simulink model "Robot_Eye_Control"  (R2016b)
settings: Solver=ode1  StartTime=0.0  StopTime=Inf  FixedStep=0.001  RelTol=1e-3
PostLoadFcn:
  | , if any(exist('dsrtsu_mdlpostloadfcn', 'file') == [2, 3, 6]), try dsrtsu_mdlpostloadfcn('Execute', bdroot); catch fprintf('Error in PostLoadFcn (dsrtsu_mdlpostloadfcn) for model "%s":\n %s\n', bdroot, lasterr); end, end,
libraries: simulink x4, rtiethernetlib x4, dspstat3 x3, rti1202serlib x2
settings Model: DSRTSU_INTERNAL_RTI_VER=490  DSRTSU_INTERNAL_RTI_TYPE=rti1202  DSRTSU_INTERNAL_RTIFPGA=80  Creator=labuser  LastModifiedBy=labuser
settings OptimizationCC: BlockReduction=off  ConditionallyExecuteInputs=off  OptimizeBlockIOStorage=off  BufferReuse=off  GlobalBufferReuse=off  ExpressionFolding=off  LocalBlockOutputs=off
settings HardwareCC: ProdBitPerPointer=32  ProdBitPerSizeT=32  ProdBitPerPtrDiffT=32  ProdLargestAtomicInteger=Integer  ProdEndianess=BigEndian  ProdWordSize=32  ProdHWDeviceType=Custom Processor->Custom  TargetIntDivRoundTo=Zero  TargetEndianess=BigEndian  TargetHWDeviceType=Custom Processor->Custom
settings RTWCC: SystemTargetFile=rti1202.tlc  MakeCommand=make_rti  TemplateMakefile=rti1202.tmf  Description=dSPACE DS1202 Hardware Platform
settings STFCustomTargetCC: ParMdlRefBuildCompliant=on  GRTInterface=off  SystemTargetFile=rti1202.tlc
settings GRTTargetCC: TargetLangStandard=C89/C90 (ANSI)  CompOptLevelCompliant=off  ConcurrentExecutionCompliant=off  CombineOutputUpdateFcns=off  MatFileLogging=off  CPPClassGenCompliant=off  UseToolchainInfoCompliant=off
settings ConfigComp: CovMetricSettings=dswe

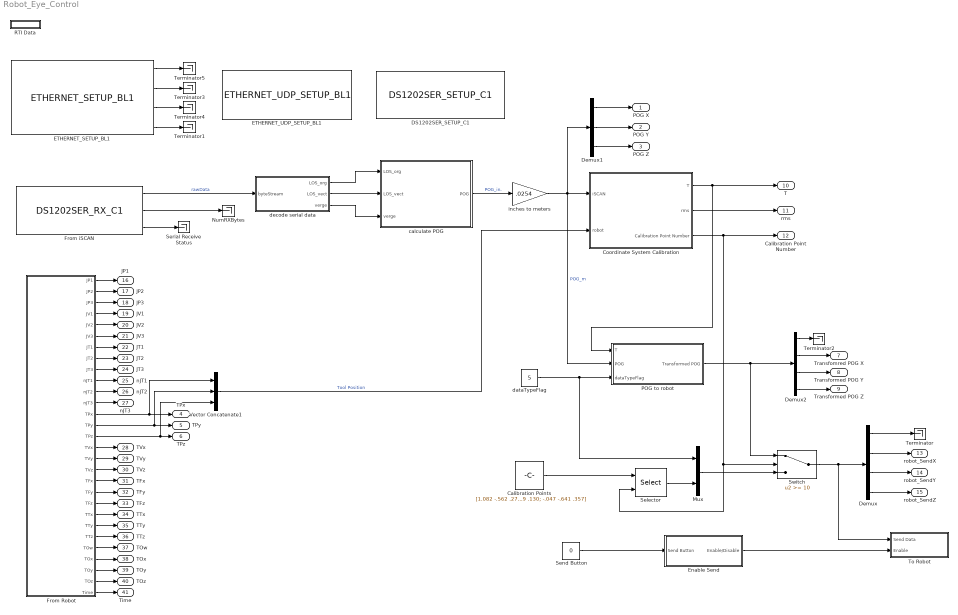
== system Robot_Eye_Control ==
  Calibration Points : Constant  Value=[1.082 -.562 .273; .898 -.561 .225; .758 -.729 .310; .477 -.680 .405; .392 -.487 .317; .510 -.267 .364; .659 -.237 .180; .924 -.322 .241; .813 -.527 .371; .567 -.539 .130; -.047 -.641 .357]  VectorParams1D=off
  Coordinate System Calibration : Subsystem
  DS1202SER_SETUP_C1 : rti1202serlib/DS1202SER_SETUP_C1  Reserved1=[]  Reserved2=[]  Reserved3=[]  Reserved4=[]  DSProperties=struct('RTI',struct('Version',uint32(2),'IOBoardType',{{'DS1202','SER'}},'SlaveProcessor','NONE','BlockType',struct('isSLSource',uint8(0),'isSLSink',uint8(0),'isHWSource',uint8(0),'isHWSink',uint8(0),'isSetup',uint8(1),'isInline',uint8(1),'isNonInline',uint8(0),'isInterrupt',uint8(0),'isChannelwise',uint8(1)),'UnitType','GENSER','Identifier','SETUP','DialogType','ML','BlockSet','NONE'))  RTIBlockInterface=struct('BlockName',struct('Token',{{'DS1202SER_SETUP_C'}},'BlockParam',{{'ChannelNo'}}),'BlockDisplay',{{['Serial Setup'],'center'}},'IconTransparency','off','ParameterTunableNames',{{}},'InitLevel',1,'DialogFcn','guigensersetup','MaskDescription',['To set the global specifications for the UART interface.'])  RTIBlockParameters=struct('ParityMode',{{1,'OFF',[1 5]}},'TransceiverMode',{{[1;1],'OFF',[]}},'QuartzFrequency',{{'160000000','OFF',[]}},'BoardNo',{{1,'ON',[1 1]}},'ChannelNo',{{1,'ON',[1 2]}},'ChannelNumOf',{{2,'OFF',[]}},'BaudRate',{{'115200','OFF',[]}},'DataBitsNumOf',{{4,'OFF',[1 4]}},'StopBitsNumOf',{{1,'OFF',[1 3]}},'ReceiveIntLevelUart',{{4,'OFF',[1 4]}},'AutoflowMode',{{0,'OFF',[]}},'FifoSize',{{'1024','OFF',[]}},'ReceiveIntLevelFifo',{{0,'OFF',[]}},'FifoOverrunMode',{{2,'OFF',[]}},'FifoBlockSize',{{'16','OFF',[]}},'TermMode',{{1,'OFF',[]}},'TLCFileName',{{'rtigensersetup','OFF',[]}})  RTISFcnParameters=struct('BoardNo','double','ChannelNo','double','ChannelNumOf','double','BaudRate','double','DataBitsNumOf','double','StopBitsNumOf','double','ParityMode','double','TransceiverMode','double','ReceiveIntLevelUart','double','AutoflowMode','double','FifoSize','double','ReceiveIntLevelFifo','double','FifoBlockSize','double','TermMode','double','QuartzFrequency','double','TLCFileName','char')  RTIBlockParaDefault=struct('ParityMode',1,'TransceiverMode',[1;1],'QuartzFrequency',160000000,'BoardNo',1,'ChannelNo',1,'ChannelNumOf',2,'BaudRate',115200,'DataBitsNumOf',4,'StopBitsNumOf',1,'ReceiveIntLevelUart',4,'AutoflowMode',0,'FifoSize',64,'ReceiveIntLevelFifo',0,'FifoOverrunMode',1,'FifoBlockSize',0,'TermMode',1,'TLCFileName','rtigensersetup')
  Demux : Demux
  Demux1 : Demux  Outputs=3
  Demux2 : Demux
  ETHERNET_SETUP_BL1 : rtiethernetlib/ETHERNET_SETUP_BL1  DSProperties=struct('RTI',struct('Version',uint32(2),'BlockType',struct('isSLSource',uint8(0),'isSLSink',uint8(0),'isHWSource',uint8(0),'isHWSink',uint8(0),'isSetup',uint8(1),'isInline',uint8(1),'isNonInline',uint8(0),'isInterrupt',uint8(0),'isChannelwise',uint8(0)),'IOBoardType','DSETHERNET','UnitType','ETHERNET','Identifier','SETUP','DialogType','ML','BlockSet','RTIETHERNET','SlaveProcessor','NONE'))  RTIBlockInterface=struct('OutputPortsWidth',int32([2 1 1 4]),'OutputPortsActive',[1 1 1 1],'OutputPortsName',{{['Link Status'],['Watchdog Status'],['DHCP Status'],['Local IP']}},'OutputPortsDataType',{{'SS_UINT32','SS_UINT32','SS_UINT32','SS_UINT8'}},'InitLevel',3,'IconTransparency','on','BlockDisplay',{{['Ethernet Setup\n\nLocal IP: By DHCP Server'],'left'}},'DialogFcn','rtiethernetsetupgui','BlockName',struct('Token',{{'ETHERNET_SETUP_BL1'}}))  RTIBlockParameters=struct('DHCPserverMode',{{1,'OFF',[0 1]}},'LocalIpNum1',{{'137','OFF',[0 255]}},'LocalIpNum2',{{'148','OFF',[0 255]}},'LocalIpNum3',{{'205','OFF',[0 255]}},'LocalIpNum4',{{'167','OFF',[0 255]}},'SubnetMaskNum1',{{'255','OFF',[0 255]}},'SubnetMaskNum2',{{'255','OFF',[0 255]}},'SubnetMaskNum3',{{'254','OFF',[0 255]}},'SubnetMaskNum4',{{'0','OFF',[0 255]}},'GatewayNum1',{{'0','OFF',[0 255]}},'GatewayNum2',{{'0','OFF',[0 255]}},'GatewayNum3',{{'0','OFF',[0 255]}},'GatewayNum4',{{'0','OFF',[0 255]}},'LinkStatusOutPortMode',{{1,'OFF',[0 1]}},'NumOfEthConnectors',{{2,'ON',[1 16]}},'WatchdogStatusOutPortMode',{{1,'OFF',[0 1]}},'LocalIpOutPortMode',{{1,'OFF',[0 1]}},'IpAndSubmaskCheck',{{int32(0),'OFF',[0 1]}},'TLCFileName',{{'rtiethernetsetup','OFF',[]}})  RTISFcnParameters=struct('DHCPserverMode','int32','LocalIpNum1','uint8','LocalIpNum2','uint8','LocalIpNum3','uint8','LocalIpNum4','uint8','SubnetMaskNum1','uint8','SubnetMaskNum2','uint8','SubnetMaskNum3','uint8','SubnetMaskNum4','uint8','GatewayNum1','uint8','GatewayNum2','uint8','GatewayNum3','uint8','GatewayNum4','uint8','LinkStatusOutPortMode','int32','NumOfEthConnectors','int32','WatchdogStatusOutPortMode','int32','LocalIpOutPortMode','int32','TLCFileName','char')  RTIBlockParaDefault=struct('DHCPserverMode',0,'LocalIpNum1',192,'LocalIpNum2',168,'LocalIpNum3',140,'LocalIpNum4',6,'SubnetMaskNum1',255,'SubnetMaskNum2',255,'SubnetMaskNum3',255,'SubnetMaskNum4',0,'GatewayNum1',0,'GatewayNum2',0,'GatewayNum3',0,'GatewayNum4',0,'LinkStatusOutPortMode',1,'NumOfEthConnectors',3,'WatchdogStatusOutPortMode',0,'LocalIpOutPortMode',0,'IpAndSubmaskCheck',1,'TLCFileName','rtiethernetsetup')
  ETHERNET_UDP_SETUP_BL1 : rtiethernetlib/ETHERNET_UDP_SETUP_BL1  DSProperties=struct('RTI',struct('Version',uint32(2),'BlockType',struct('isSLSource',uint8(1),'isSLSink',uint8(1),'isHWSource',uint8(0),'isHWSink',uint8(0),'isSetup',uint8(0),'isInline',uint8(1),'isNonInline',uint8(0),'isInterrupt',uint8(0),'isChannelwise',uint8(0)),'IOBoardType','DSETHERNET','UnitType','UDP','Identifier','SETUPUDP','DialogType','ML','BlockSet','RTIETHERNET','SlaveProcessor','NONE'))  RTIBlockInterface=struct('OutputPortsWidth',int32(2),'OutputPortsActive',0,'OutputPortsName',{{['RX Dropped Frames']}},'OutputPortsDataType',{{'SS_DOUBLE'}},'InputPortsWidth',int32([4 1]),'InputPortsActive',int32([0 0]),'InputPortsName',{{['RX Remote IP Filter'],['RX Remote Port Filter']}},'InputPortsDataType',{{'SS_UINT8','SS_UINT16'}},'RWork',{{{'RX_DROPPED_FRAMES',uint32(2)}}},'InitLevel',3,'IconTransparency','on','BlockDisplay',{{['Ethernet UDP/IP\nSetup\n\nSocket ID: 0'],'center'}},'DialogFcn','rtiethernetsetupudpgui','BlockName',struct('Token',{{'ETHERNET_UDP_SETUP_BL1'}}))  RTIBlockParameters=struct('SocketId',{{0,'OFF',[]}},'EnableSocketBind',{{1,'OFF',[0 1]}},'AcceptAnyRxRemoteIp',{{1,'OFF',[0 1]}},'RxRemoteIpNum1',{{'172','OFF',[0 255]}},'RxRemoteIpNum2',{{'20','OFF',[0 255]}},'RxRemoteIpNum3',{{'41','OFF',[0 255]}},'RxRemoteIpNum4',{{'226','OFF',[0 255]}},'EnableDynamicRxRemoteIpFilter',{{0,'OFF',[0 1]}},'AcceptAnyRxRemotePort',{{1,'OFF',[0 1]}},'RxRemotePort',{{'9930','OFF',[1 65535]}},'EnableDynamicRxRemotePortFilter',{{0,'OFF',[0 1]}},'TxRemoteIpNum1',{{'137','OFF',[0 255]}},'TxRemoteIpNum2',{{'148','OFF',[0 255]}},'TxRemoteIpNum3',{{'204','OFF',[0 255]}},'TxRemoteIpNum4',{{'55','OFF',[0 255]}},'TxRemotePort',{{'9930','OFF',[1 65535]}},'SpecifyLocalPort',{{1,'OFF',[0 1]}},'LocalPort',{{'9931','OFF',[1 65535]}},'InterruptMode',{{0,'OFF',[0 1]}},'RxDroppedFramesOutPortMode',{{0,'OFF',[0 1]}},'RemoteIpNumCheck',{{0,'OFF',[0 1]}},'RemotePortCheck',{{0,'OFF',[0 1]}},'LocalPortCheck',{{1,'OFF',[0 1]}},'DHCPserverModeEnabled',{{0,'OFF',[0 1]}},'TLCFileName',{{'rtiethernetsetupudp','OFF',[]}})  RTISFcnParameters=struct('SocketId','double','EnableSocketBind','int32','AcceptAnyRxRemoteIp','int32','RxRemoteIpNum1','uint8','RxRemoteIpNum2','uint8','RxRemoteIpNum3','uint8','RxRemoteIpNum4','uint8','EnableDynamicRxRemoteIpFilter','int32','AcceptAnyRxRemotePort','int32','RxRemotePort','uint16','EnableDynamicRxRemotePortFilter','int32','TxRemoteIpNum1','uint8','TxRemoteIpNum2','uint8','TxRemoteIpNum3','uint8','TxRemoteIpNum4','uint8','TxRemotePort','uint16','SpecifyLocalPort','int32','LocalPort','uint16','InterruptMode','int32','RxDroppedFramesOutPortMode','int32','DHCPserverModeEnabled','int32','TLCFileName','char')  RTIBlockParaDefault=struct('SocketId',-1,'EnableSocketBind',1,'AcceptAnyRxRemoteIp',1,'RxRemoteIpNum1',0,'RxRemoteIpNum2',0,'RxRemoteIpNum3',0,'RxRemoteIpNum4',0,'EnableDynamicRxRemoteIpFilter',0,'AcceptAnyRxRemotePort',1,'RxRemotePort',49002,'EnableDynamicRxRemotePortFilter',0,'TxRemoteIpNum1',0,'TxRemoteIpNum2',0,'TxRemoteIpNum3',0,'TxRemoteIpNum4',0,'TxRemotePort',49002,'SpecifyLocalPort',0,'LocalPort',49001,'InterruptMode',0,'RxDroppedFramesOutPortMode',0,'RemoteIpNumCheck',0,'RemotePortCheck',0,'LocalPortCheck',0,'DHCPserverModeEnabled',0,'TLCFileName','rtiethernetsetupudp')
  Enable Send : Subsystem
  From Robot : Subsystem
  From iSCAN : rti1202serlib/DS1202SER_RX_C1  Reserved1=[]  Reserved2=[]  Reserved3=[]  Reserved4=[]  DSProperties=struct('RTI',struct('IOBoardType',{{'DS1202','SER'}},'SlaveProcessor','NONE','Version',uint32(1),'BlockType',struct('isSLSource',uint8(1),'isSLSink',uint8(1),'isHWSource',uint8(0),'isHWSink',uint8(1),'isSetup',uint8(0),'isInline',uint8(1),'isNonInline',uint8(0),'isInterrupt',uint8(0),'isChannelwise',uint8(1)),'UnitType','GENSER','Identifier','RECEIVE','DialogType','ML','BlockSet','NONE'))  RTIBlockInterface=struct('BlockName',struct('Token',{{'DS1202SER_RX_C'}},'BlockParam',{{'ChannelNo'}}),'InputPortsWidth',int32(1),'InputPortsActive',0,'InputPortsDataType',{{'SS_UINT32'}},'InputPortsName',{{'NumBytes'}},'OutputPortsWidth',int32([16 1 1]),'OutputPortsActive',[1 1 1],'OutputPortsDataType',{{'SS_UINT8','SS_UINT32','SS_INT32'}},'OutputPortsName',{{'RXBytes','NumRXBytes','Status'}},'BlockDisplay',{{['Serial Receive'],'center'}},'IconTransparency','on','ParameterTunableNames',{{}},'InitLevel',2,'DialogFcn','guigenserreceive','MaskDescription',['To read data from the UART SW FIFO.'])  RTIBlockParameters=struct('BoardNo',{{1,'ON',[1 1]}},'ChannelNo',{{1,'ON',[1 2]}},'ChannelNumOf',{{2,'OFF',[]}},'ReceptionDataMode',{{1,'OFF',[]}},'ParamTunableMode',{{2,'OFF',[]}},'BytesRefNumOfT',{{'1','OFF',[1 inf]}},'BytesRefNumOfNT',{{'16','OFF',[1 inf]}},'BytesRefNumOfMax',{{'1','OFF',[1 inf]}},'BytesRefNumOfMode',{{1,'OFF',[]}},'BytesActNumOfMode',{{1,'OFF',[]}},'ReceptionStatusMode',{{1,'OFF',[]}},'FifoSizeDefault',{{64,'OFF',[]}},'TLCFileName',{{'rtigenserreceive','OFF',[]}})  RTISFcnParameters=struct('BoardNo','double','ChannelNo','double','ChannelNumOf','double','ReceptionDataMode','double','ParamTunableMode','double','BytesRefNumOfT','double','BytesRefNumOfNT','double','BytesRefNumOfMax','double','BytesRefNumOfMode','double','BytesActNumOfMode','double','ReceptionStatusMode','double','TLCFileName','char')  RTIBlockParaDefault=struct('BoardNo',1,'ChannelNo',1,'ChannelNumOf',2,'ReceptionDataMode',1,'ParamTunableMode',1,'BytesRefNumOfT',1,'BytesRefNumOfNT',1,'BytesRefNumOfMax',1,'BytesRefNumOfMode',0,'BytesActNumOfMode',1,'ReceptionStatusMode',1,'FifoSizeDefault',64,'TLCFileName','rtigenserreceive')
  Mux : Mux  Inputs=2
  NumRXBytes : Terminator
  POG to robot : Subsystem
  RTI Data : Subsystem  Tag=struct('RTIDataServer',struct('RTIDataServerVs','2','RTIModelDescription','struct(''main'',''Robot_Eye_Control'',''sub'','''',''isMp'',0)'))  LoadFcn="if exist('rtidc'), try,  rtidc('DataHostBlockClbLoad', gcbh); catch, disp(['Warning: ''LoadFcn'' for RTI Data block failed: ' lasterr]); end, end,"  mask(RTI_DATA_HOST){}
      mask help:
      | RTI Data Block.
      | This block is used by RTI to store internal model-dependent data.
      | Please keep this block on the root level of the model. Deleting this block will result in data loss.
      |
      | NEVER DELETE OR COPY THIS BLOCK!
      settings: CopyFcn="if exist('rtidc'), try,  rtidc('DataHostBlockClbCopy', gcbh); catch, disp(['Warning: ''CopyFcn'' for RTI Data block failed: ' lasterr]); end, end,"  DeleteFcn="if exist('rtidc'), try,  rtidc('DataHostBlockClbDelete', gcbh); catch, disp(['Warning: ''DeleteFcn'' for RTI Data block failed: ' lasterr]); end, end,"  ModelCloseFcn="if exist('rtidc'), try,  rtidc('DataHostBlockClbModelClose', gcbh); catch, disp(['Warning: ''ModelCloseFcn'' for RTI Data block failed: ' lasterr]); end, end,"  PreSaveFcn="if exist('rtidc'), try,  rtidc('DataHostBlockClbPreSave', gcbh); catch, disp(['Warning: ''PreSaveFcn'' for RTI Data block failed: ' lasterr]); end, end,"  PostSaveFcn="if exist('rtidc'), try,  rtidc('DataHostBlockClbPostSave', gcbh); catch, disp(['Warning: ''PostSaveFcn'' for RTI Data block failed: ' lasterr]); end, end,"  NameChangeFcn="if exist('rtidc'), try,  rtidc('DataHostBlockClbNameChange', gcbh); catch, disp(['Warning: ''NameChangeFcn'' for RTI Data block failed: ' lasterr]); end, end,"
      mask Help:
      | RTI Data Block.
      | This block is used by RTI to store internal model-dependent data.
      | Please keep this block on the root level of the model. Deleting this block will result in data loss.
      | 
      | NEVER DELETE OR COPY THIS BLOCK!
      mask Display:
      | text(0.5, 0.5, 'RTI Data', 'HorizontalAlignment', 'center');
      | plot([1 0]);
  Selector : Selector  NumberOfDimensions=2  IndexMode=Zero-based  InputPortWidth=3  IndexOptions=Index vector (port),Select all  Indices=[1 3],1  OutputSizes=1,1
  Send Button : Constant  Value=0
  Serial Receive Status : Terminator
  Switch : Switch  Threshold=10
  Terminator{,1..5} (6 alike) : Terminator
  To Robot : Subsystem
  Vector Concatenate1 : Concatenate  NumInputs=3  Mode=Multidimensional array  ConcatenateDimension=2
  calculate POG : Subsystem
  dataTypeFlag : Constant  Value=5
  decode serial data : MATLAB Function  TreatAsAtomicUnit=on
  inches to meters : Gain  Gain=.0254
  POG X : Outport
  POG Y : Outport  Port=2
  POG Z : Outport  Port=3
  TPx : Outport  Port=4
  TPy : Outport  Port=5
  TPz : Outport  Port=6
  Transfomred POG X : Outport  Port=7
  Transformed POG Y : Outport  Port=8
  Transformed POG Z : Outport  Port=9
  T : Outport  Port=10
  rms : Outport  Port=11
  Calibration Point Number : Outport  Port=12
  robot_SendX : Outport  Port=13
  robot_SendY : Outport  Port=14
  robot_SendZ : Outport  Port=15
  JP1 : Outport  Port=16
  JP2 : Outport  Port=17
  JP3 : Outport  Port=18
  JV1 : Outport  Port=19
  JV2 : Outport  Port=20
  JV3 : Outport  Port=21
  JT1 : Outport  Port=22
  JT2 : Outport  Port=23
  JT3 : Outport  Port=24
  nJT1 : Outport  Port=25
  nJT2 : Outport  Port=26
  nJT3 : Outport  Port=27
  TVx : Outport  Port=28
  TVy : Outport  Port=29
  TVz : Outport  Port=30
  TFx : Outport  Port=31
  TFy : Outport  Port=32
  TFz : Outport  Port=33
  TTx : Outport  Port=34
  TTy : Outport  Port=35
  TTz : Outport  Port=36
  TOw : Outport  Port=37
  TOx : Outport  Port=38
  TOy : Outport  Port=39
  TOz : Outport  Port=40
  Time : Outport  Port=41
  wires:
  From iSCAN/2 -> NumRXBytes/1
  From iSCAN/3 -> Serial Receive Status/1
  From iSCAN/1 -> decode serial data/1(byteStream)  "rawData"
  ETHERNET_SETUP_BL1/3 -> Terminator4/1
  ETHERNET_SETUP_BL1/4 -> Terminator1/1
  Vector Concatenate1/1 -> Coordinate System Calibration/2(robot)  "Tool Position"
  Coordinate System Calibration/3(Calibration Point Number) -> Switch/2, Selector/2, Calibration Point Number/1
  Coordinate System Calibration/2(rms) -> rms/1
  Coordinate System Calibration/1(T) -> POG to robot/1(T), T/1
  From Robot/13(TPx) -> Vector Concatenate1/1, TPx/1
  From Robot/14(TPy) -> Vector Concatenate1/2, TPy/1
  From Robot/15(TPz) -> Vector Concatenate1/3, TPz/1
  From Robot/1(JP1) -> JP1/1
  From Robot/2(JP2) -> JP2/1
  From Robot/3(JP3) -> JP3/1
  From Robot/29(Time) -> Time/1
  From Robot/28(TOz) -> TOz/1
  From Robot/27(TOy) -> TOy/1
  From Robot/26(TOx) -> TOx/1
  From Robot/25(TOw) -> TOw/1
  From Robot/24(TTz) -> TTz/1
  From Robot/23(TTy) -> TTy/1
  From Robot/22(TTx) -> TTx/1
  From Robot/21(TFz) -> TFz/1
  From Robot/20(TFy) -> TFy/1
  From Robot/19(TFx) -> TFx/1
  From Robot/18(TVz) -> TVz/1
  From Robot/17(TVy) -> TVy/1
  From Robot/16(TVx) -> TVx/1
  From Robot/12(nJT3) -> nJT3/1
  From Robot/11(nJT2) -> nJT2/1
  From Robot/10(nJT1) -> nJT1/1
  From Robot/9(JT3) -> JT3/1
  From Robot/8(JT2) -> JT2/1
  From Robot/7(JT1) -> JT1/1
  From Robot/6(JV3) -> JV3/1
  From Robot/5(JV2) -> JV2/1
  From Robot/4(JV1) -> JV1/1
  decode serial data/2(LOS_vect) -> calculate POG/2(LOS_vect)
  decode serial data/1(LOS_org) -> calculate POG/1(LOS_org)
  decode serial data/3(verge) -> calculate POG/3(verge)
  dataTypeFlag/1 -> Mux/1, POG to robot/3(dataTypeFlag)
  Enable Send/1(Enable/Disable) -> To Robot/2(Enable)
  Send Button/1 -> Enable Send/1(Send Button)
  Switch/1 -> To Robot/1(Send Data), Demux/1
  POG to robot/1(Transformed POG) -> Demux2/1, Switch/1
  Mux/1 -> Switch/3
  Selector/1 -> Mux/2
  Calibration Points/1 -> Selector/1
  Demux/1 -> Terminator/1
  Demux/2 -> robot_SendX/1
  Demux/4 -> robot_SendZ/1
  Demux/3 -> robot_SendY/1
  calculate POG/1(POG) -> inches to meters/1  "POG_in."
  inches to meters/1 -> Demux1/1, POG to robot/2(POG), Coordinate System Calibration/1(iSCAN)  "POG_m"
  Demux1/3 -> POG Z/1
  Demux1/2 -> POG Y/1
  Demux1/1 -> POG X/1
  Demux2/1 -> Terminator2/1
  Demux2/2 -> Transfomred POG X/1
  Demux2/3 -> Transformed POG Y/1
  Demux2/4 -> Transformed POG Z/1
  ETHERNET_SETUP_BL1/1 -> Terminator5/1
  ETHERNET_SETUP_BL1/2 -> Terminator3/1

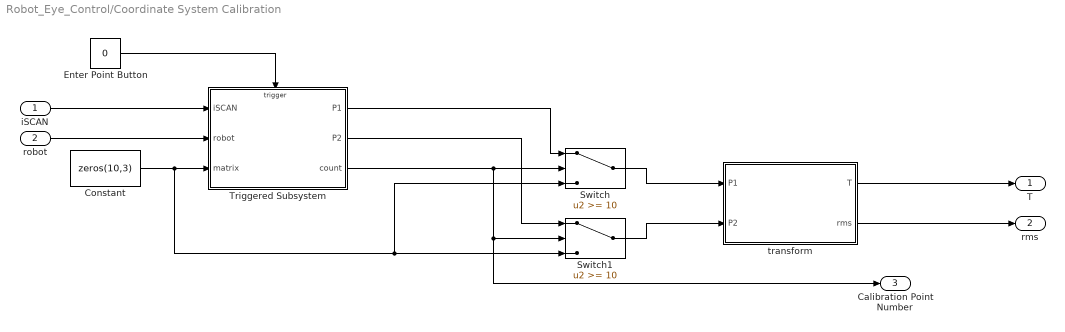
== system Robot_Eye_Control/Coordinate System Calibration ==
  iSCAN : Inport
  robot : Inport  Port=2
  Constant : Constant  Value=zeros(10,3)  VectorParams1D=off
  Enter Point Button : Constant  Value=0  VectorParams1D=off
  Switch : Switch  Threshold=10
  Switch1 : Switch  Threshold=10
  Triggered Subsystem : Subsystem  TreatAsAtomicUnit=on
  transform : MATLAB Function  TreatAsAtomicUnit=on
  T : Outport
  rms : Outport  Port=2
  Calibration Point Number : Outport  Port=3
  wires:
  Enter Point Button/1 -> Triggered Subsystem/Trigger
  iSCAN/1 -> Triggered Subsystem/1(iSCAN)
  robot/1 -> Triggered Subsystem/2(robot)
  Triggered Subsystem/3(count) -> Calibration Point Number/1, Switch1/2, Switch/2
  Triggered Subsystem/1(P1) -> Switch/1
  Triggered Subsystem/2(P2) -> Switch1/1
  Constant/1 -> Switch/3, Switch1/3, Triggered Subsystem/3(matrix)
  Switch/1 -> transform/1(P1)
  Switch1/1 -> transform/2(P2)
  transform/1(T) -> T/1
  transform/2(rms) -> rms/1

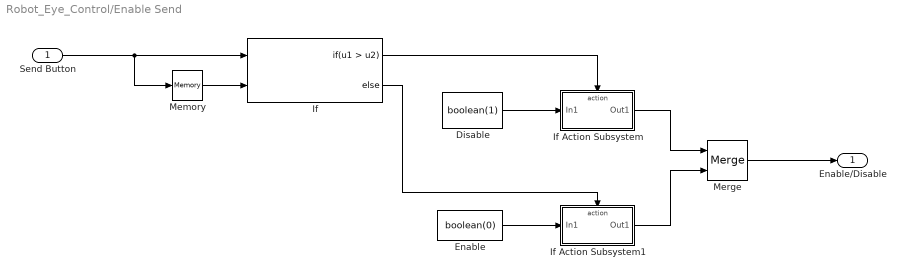
== system Robot_Eye_Control/Enable Send ==
  Send Button : Inport
  Disable : Constant  Value=boolean(1)
  Enable : Constant  Value=boolean(0)
  If : If  NumInputs=2  IfExpression=u1 > u2
  If Action Subsystem : Subsystem  TreatAsAtomicUnit=on
  If Action Subsystem1 : Subsystem  TreatAsAtomicUnit=on
  Memory : Memory
  Merge : Merge
  Enable/Disable : Outport
  wires:
  If Action Subsystem1/1(Out1) -> Merge/2
  If/1 -> If Action Subsystem/Action
  If/2 -> If Action Subsystem1/Action
  Send Button/1 -> Memory/1, If/1
  Enable/1 -> If Action Subsystem1/1(In1)
  Memory/1 -> If/2
  Merge/1 -> Enable/Disable/1
  Disable/1 -> If Action Subsystem/1(In1)
  If Action Subsystem/1(Out1) -> Merge/1

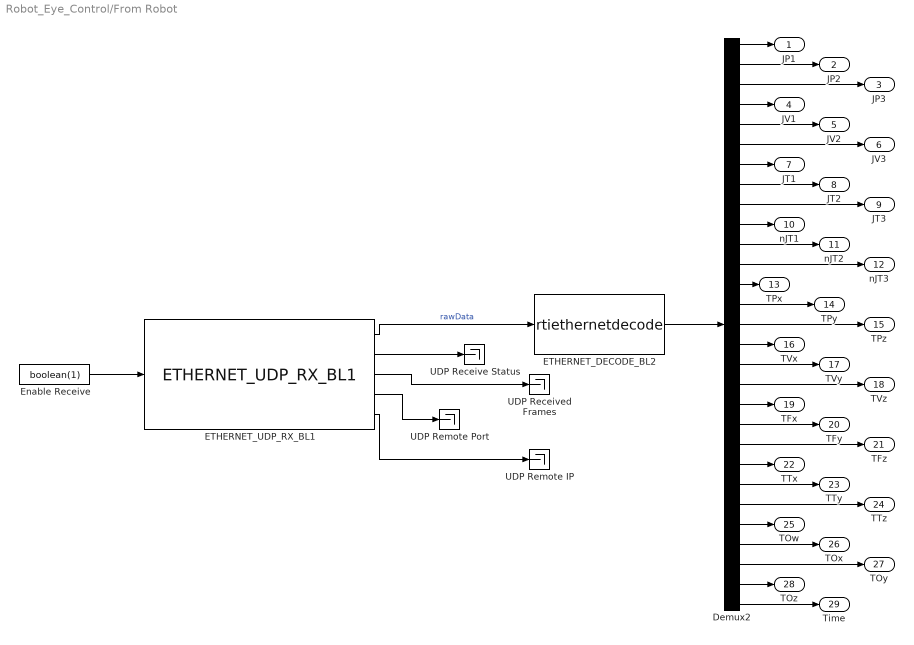
== system Robot_Eye_Control/From Robot ==
  Demux2 : Demux  Outputs=29
  ETHERNET_DECODE_BL2 : S-Function  FunctionName=rtiethernetdecode  Parameters=byteordering,offset,auto_offset,datatype,one_datatype,sampletime  SFunctionDeploymentMode=off  EnableBusSupport=off  mask(Ethernet Decode){byteordering=Little endian (Intel), offset=[0], auto_offset=on, datatype=[9 9 9 9 9 9 9 9 9 9 9 9 9 9 9 9 9 9 9 9 9 9 9 9 9 9 9 9 3], one_datatype=off, sampletime=.002}
      mask prompts: byteordering "Byte ordering:"; offset "Offset (bytes):"; auto_offset "Auto offset"; one_datatype "One datatype only"
      mask help:
      | Converts a byte input data stream into the specified datatypes on the output port.
      |
      | Datatype codes:
      | BOOLEAN:  1   //   INT8:      2   //   UINT8:    3
      | INT16  :     4   //   UINT16:  5   //   INT32:     6
      | UINT32 :    7   //   FLOAT:    8   //   DOUBLE:  9
      mask Help: To get further information on this block, refer to the RTI Ethernet blockset documentation.
      mask TypeOptions byteordering: Big endian (Motorola) | Little endian (Intel)
      mask Callback auto_offset: rtiethernetfcnlib('EnableEnDecodeGuiControl', gcbh, 'auto_offset', 2)
      mask Display: text(0.5,0.5, 'Ethernet\nDecode', 'HorizontalAlignment', 'center')
  ETHERNET_UDP_RX_BL1 : rtiethernetlib/ETHERNET_UDP_RX_BL1  DSProperties=struct('RTI',struct('Version',uint32(1),'BlockType',struct('isSLSource',uint8(1),'isSLSink',uint8(1),'isHWSource',uint8(0),'isHWSink',uint8(1),'isSetup',uint8(0),'isInline',uint8(1),'isNonInline',uint8(0),'isInterrupt',uint8(0),'isChannelwise',uint8(0)),'IOBoardType','DSETHERNET','UnitType','UDP','Identifier','RXUDP','DialogType','ML','BlockSet','RTIETHERNET','SlaveProcessor','NONE'))  RTIBlockInterface=struct('OutputPortsWidth',int32([232 1 1 1 4 1]),'OutputPortsActive',[1 1 1 0 1 1],'OutputPortsName',{{'Data','Status',['Received Frames'],['Received Bytes'],['Remote IP'],['Remote Port']}},'OutputPortsDataType',{{'SS_UINT8','SS_UINT32','SS_DOUBLE','SS_UINT32','SS_UINT8','SS_UINT16'}},'InputPortsWidth',int32(1),'InputPortsActive',1,'InputPortsName',{{'Enable'}},'InputPortsDataType',{{'SS_BOOLEAN'}},'RWork',{{{'RECEIVED_FRAMES',uint32(1)}}},'InitLevel',3,'IconTransparency','on','BlockDisplay',{{['Ethernet UDP/IP\nRX\n\nSocket ID: 0'],'center'}},'DialogFcn','rtiethernetrxudpgui','BlockName',struct('Token',{{'ETHERNET_UDP_RX_BL1'}}))  RTIBlockParameters=struct('SocketIdIndex',{{2,'OFF',[1 2]}},'SocketId',{{0,'OFF',[-1 inf]}},'RemoteIp',{{['<NOT AVAILABLE>'],'OFF',[]}},'RemotePort',{{['<NOT AVAILABLE>'],'OFF',[]}},'LocalPort',{{9931,'OFF',[]}},'FrameSize',{{'232','OFF',[1 65507]}},'EnableVariableFrameSize',{{0,'OFF',[0 1]}},'VariableFrameSizeMode',{{1,'OFF',[1 2]}},'InterruptMode',{{0,'OFF',[0 1]}},'RemoteIpOutPortMode',{{1,'OFF',[0 1]}},'RemotePortOutPortMode',{{1,'OFF',[0 1]}},'TLCFileName',{{'rtiethernetrxudp','OFF',[]}})  RTISFcnParameters=struct('SocketIdIndex','int32','SocketId','double','FrameSize','uint16','EnableVariableFrameSize','int32','VariableFrameSizeMode','int32','InterruptMode','int32','RemoteIpOutPortMode','int32','RemotePortOutPortMode','int32','TLCFileName','char')  RTIBlockParaDefault=struct('SocketIdIndex',1,'SocketId',-1,'RemoteIp',['<NOT AVAILABLE>'],'RemotePort',['<NOT AVAILABLE>'],'LocalPort',['<NOT AVAILABLE>'],'FrameSize',1024,'EnableVariableFrameSize',0,'VariableFrameSizeMode',1,'InterruptMode',0,'RemoteIpOutPortMode',0,'RemotePortOutPortMode',0,'TLCFileName','rtiethernetrxudp')
  Enable Receive : Constant  Value=boolean(1)
  UDP Receive Status : Terminator
  UDP Received Frames : Terminator
  UDP Remote IP : Terminator
  UDP Remote Port : Terminator
  JP1 : Outport
  JP2 : Outport  Port=2
  JP3 : Outport  Port=3
  JV1 : Outport  Port=4
  JV2 : Outport  Port=5
  JV3 : Outport  Port=6
  JT1 : Outport  Port=7
  JT2 : Outport  Port=8
  JT3 : Outport  Port=9
  nJT1 : Outport  Port=10
  nJT2 : Outport  Port=11
  nJT3 : Outport  Port=12
  TPx : Outport  Port=13
  TPy : Outport  Port=14
  TPz : Outport  Port=15
  TVx : Outport  Port=16
  TVy : Outport  Port=17
  TVz : Outport  Port=18
  TFx : Outport  Port=19
  TFy : Outport  Port=20
  TFz : Outport  Port=21
  TTx : Outport  Port=22
  TTy : Outport  Port=23
  TTz : Outport  Port=24
  TOw : Outport  Port=25
  TOx : Outport  Port=26
  TOy : Outport  Port=27
  TOz : Outport  Port=28
  Time : Outport  Port=29
  wires:
  ETHERNET_UDP_RX_BL1/2 -> UDP Receive Status/1
  ETHERNET_UDP_RX_BL1/5 -> UDP Remote IP/1
  ETHERNET_UDP_RX_BL1/4 -> UDP Remote Port/1
  ETHERNET_UDP_RX_BL1/1 -> ETHERNET_DECODE_BL2/1  "rawData"
  ETHERNET_UDP_RX_BL1/3 -> UDP Received Frames/1
  Enable Receive/1 -> ETHERNET_UDP_RX_BL1/1
  Demux2/4 -> JV1/1
  Demux2/5 -> JV2/1
  Demux2/6 -> JV3/1
  Demux2/7 -> JT1/1
  Demux2/8 -> JT2/1
  Demux2/9 -> JT3/1
  Demux2/10 -> nJT1/1
  Demux2/11 -> nJT2/1
  Demux2/12 -> nJT3/1
  Demux2/14 -> TPy/1
  Demux2/15 -> TPz/1
  Demux2/16 -> TVx/1
  Demux2/17 -> TVy/1
  Demux2/18 -> TVz/1
  Demux2/19 -> TFx/1
  Demux2/20 -> TFy/1
  Demux2/21 -> TFz/1
  Demux2/22 -> TTx/1
  Demux2/23 -> TTy/1
  Demux2/24 -> TTz/1
  Demux2/1 -> JP1/1
  Demux2/2 -> JP2/1
  Demux2/3 -> JP3/1
  Demux2/25 -> TOw/1
  Demux2/26 -> TOx/1
  Demux2/27 -> TOy/1
  Demux2/28 -> TOz/1
  Demux2/29 -> Time/1
  ETHERNET_DECODE_BL2/1 -> Demux2/1
  Demux2/13 -> TPx/1

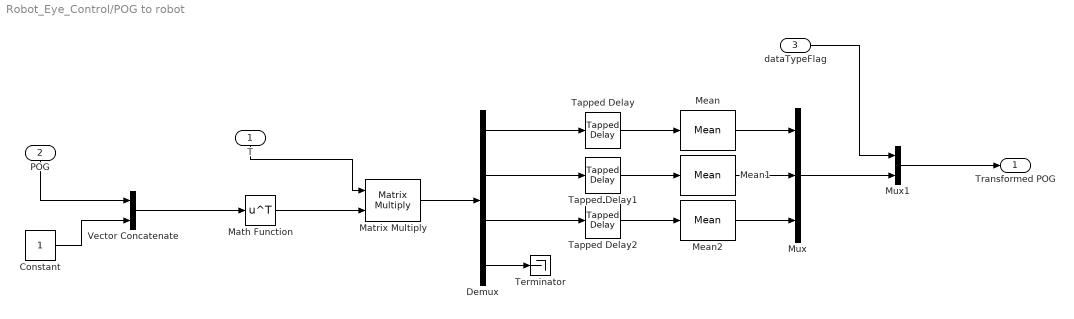
== system Robot_Eye_Control/POG to robot ==
  T : Inport
  POG : Inport  Port=2
  dataTypeFlag : Inport  Port=3
  Constant : Constant
  Demux : Demux
  Math Function : Math  Operator=transpose  SaturateOnIntegerOverflow=on
  Matrix Multiply : Product  Multiplication=Matrix(*)
  Mean : dspstat3/Mean  run=off  reset_popup=None  InputProcessing=Columns as channels (frame based)  directionMode=Each column  dimension=1  roiEnable=off  roiType=Rectangles  roiPortion=Entire ROI  roiOutput=Individual statistics for each ROI  roiFlag=off  outputDataTypeStr=Inherit: Same as accumulator  outputLastDataTypeStr=Inherit: Same as accumulator  outputMin=[]  outputMax=[]  roundingMode=Floor  overflowMode=off
  Mean1 : dspstat3/Mean  run=off  reset_popup=None  InputProcessing=Columns as channels (frame based)  directionMode=Each column  dimension=1  roiEnable=off  roiType=Rectangles  roiPortion=Entire ROI  roiOutput=Individual statistics for each ROI  roiFlag=off  outputDataTypeStr=Inherit: Same as accumulator  outputLastDataTypeStr=Inherit: Same as accumulator  outputMin=[]  outputMax=[]  roundingMode=Floor  overflowMode=off
  Mean2 : dspstat3/Mean  run=off  reset_popup=None  InputProcessing=Columns as channels (frame based)  directionMode=Each column  dimension=1  roiEnable=off  roiType=Rectangles  roiPortion=Entire ROI  roiOutput=Individual statistics for each ROI  roiFlag=off  outputDataTypeStr=Inherit: Same as accumulator  outputLastDataTypeStr=Inherit: Same as accumulator  outputMin=[]  outputMax=[]  roundingMode=Floor  overflowMode=off
  Mux : Mux  Inputs=3
  Mux1 : Mux  Inputs=2
  Tapped Delay : simulink/Discrete/Tapped Delay  vinit=0.0  samptime=-1  NumDelays=10  DelayOrder=Oldest  includeCurrent=off
  Tapped Delay1 : simulink/Discrete/Tapped Delay  vinit=0.0  samptime=-1  NumDelays=10  DelayOrder=Oldest  includeCurrent=off
  Tapped Delay2 : simulink/Discrete/Tapped Delay  vinit=0.0  samptime=-1  NumDelays=10  DelayOrder=Oldest  includeCurrent=off
  Terminator : Terminator
  Vector Concatenate : Concatenate
  Transformed POG : Outport
  wires:
  T/1 -> Matrix Multiply/1
  POG/1 -> Vector Concatenate/1
  dataTypeFlag/1 -> Mux1/1
  Vector Concatenate/1 -> Math Function/1
  Mux1/1 -> Transformed POG/1
  Matrix Multiply/1 -> Demux/1
  Demux/1 -> Tapped Delay/1
  Demux/3 -> Tapped Delay2/1
  Demux/4 -> Terminator/1
  Demux/2 -> Tapped Delay1/1
  Constant/1 -> Vector Concatenate/2
  Math Function/1 -> Matrix Multiply/2
  Tapped Delay/1 -> Mean/1
  Tapped Delay1/1 -> Mean1/1
  Tapped Delay2/1 -> Mean2/1
  Mean/1 -> Mux/1
  Mean1/1 -> Mux/2
  Mean2/1 -> Mux/3
  Mux/1 -> Mux1/2

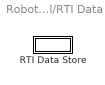
== system Robot_Eye_Control/RTI Data ==
  RTI Data Store : Subsystem  Tag="struct('public',struct('sub',struct('name',{{'Robot_Eye_Control'}},'data',{{struct('TH',struct('thTaskInfo',struct('taskType',{'TIMER','HWINT','TMRINT','SWINT','GLINT'},'tasksNumOf',{1,0,0,0,0},'srcIds',{{'TIMERA'},{},{},{},{}},'taskNames',{{['Timer Task 1']},{},{},{},{}})),'th_tc',struct('dataType','TASK','taskGroupId','','taskGroupList',{{}},'taskSchedulingPolicy','FCFS','taskType','TIMER','blkh',-1,'srcId','TIMERA','srcSgnName',['Timer A interrupt'],'srcCpuName','','taskName',['Timer Task 1  [0.001] s'],'taskNameDisplayExt','','smplTime',0.001,'smplTimeOffs',0,'hasFixedPriority',0,'priority',1,'hasFixedOvc',0,'ovcType',1,'ovcMax',1),'tc_th',struct('dataType','TASK','taskGroupId','','taskGroupList',{{}},'taskSchedulingPolicy','FCFS','taskType','TIMER','blkh',-1,'srcId','TIMERA','srcSgnName',['Timer A interrupt'],'srcCpuName','','taskName',['Timer Task 1  [0.001] s'],'taskNameDisplayExt','','smplTime',0.001,'smplTimeOffs',0,'hasFixedPriority',0,'priority',1,'hasFixedOvc',0,'ovcType',1,'ovcMax',1))}})),'private',struct('version',struct('dsVer',uint32(2)),'access',struct('modified',['22-Jan-2020 16:25:55'],'type','Model','isPerm',1)))"  mask(RTI_DATA_STORE){}
      mask help:
      | RTI Data Store Block. This block is used by RTI to store internal model dependent data. Deleting this block will result in data loss.
      |
      | NEVER DELETE, COPY, OR MODIFY THIS BLOCK!
      mask Help:
      | RTI Data Store Block. This block is used by RTI to store internal model dependent data. Deleting this block will result in data loss.
      | 
      | NEVER DELETE, COPY, OR MODIFY THIS BLOCK!
      mask Display: text(0.5, 0.5, ' ', 'HorizontalAlignment', 'center');

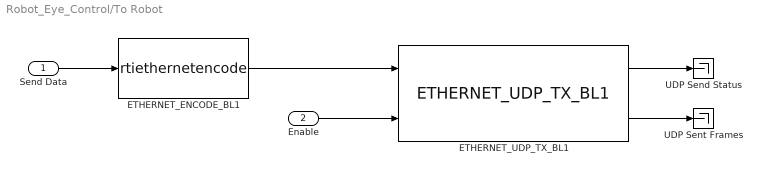
== system Robot_Eye_Control/To Robot ==
  Send Data : Inport
  Enable : Inport  Port=2
  ETHERNET_ENCODE_BL1 : S-Function  FunctionName=rtiethernetencode  Parameters=byteordering,offset,auto_offset,datatype,one_datatype,sampletime  SFunctionDeploymentMode=off  EnableBusSupport=off  mask(Ethernet Encode){byteordering=Little endian (Intel), offset=[0], auto_offset=on, datatype=[3 9 9 9], one_datatype=off, sampletime=.002}
      mask prompts: byteordering "Byte ordering:"; offset "Offset (bytes):"; auto_offset "Auto offset"; one_datatype "One datatype only"
      mask help:
      | Converts an input signal consisting of datatypes into a byte data stream on the output port.
      |
      | Datatype codes:
      | BOOLEAN:  1   //   INT8:      2   //   UINT8:    3
      | INT16  :     4   //   UINT16:  5   //   INT32:     6
      | UINT32 :    7   //   FLOAT:    8   //   DOUBLE:  9
      mask Help: To get further information on this block, refer to the RTI Ethernet blockset documentation.
      mask TypeOptions byteordering: Big endian (Motorola) | Little endian (Intel)
      mask Callback auto_offset: rtiethernetfcnlib('EnableEnDecodeGuiControl', gcbh, 'auto_offset', 2)
      mask Display: text(0.5,0.5, 'Ethernet\nEncode', 'HorizontalAlignment', 'center')
  ETHERNET_UDP_TX_BL1 : rtiethernetlib/ETHERNET_UDP_TX_BL1  DSProperties=struct('RTI',struct('Version',uint32(1),'BlockType',struct('isSLSource',uint8(1),'isSLSink',uint8(1),'isHWSource',uint8(0),'isHWSink',uint8(1),'isSetup',uint8(0),'isInline',uint8(1),'isNonInline',uint8(0),'isInterrupt',uint8(0),'isChannelwise',uint8(0)),'IOBoardType','DSETHERNET','UnitType','UDP','Identifier','TXUDP','DialogType','ML','BlockSet','RTIETHERNET','SlaveProcessor','NONE'))  RTIBlockInterface=struct('OutputPortsWidth',int32([1 1]),'OutputPortsActive',[1 1],'OutputPortsName',{{'Status',['Sent Frames']}},'OutputPortsDataType',{{'SS_UINT32','SS_DOUBLE'}},'InputPortsWidth',int32([25 1 1 4 1]),'InputPortsActive',[1 1 0 0 0],'InputPortsName',{{'Data','Enable',['Bytes to Send'],['Remote IP'],['Remote Port']}},'InputPortsDataType',{{'SS_UINT8','SS_BOOLEAN','SS_UINT32','SS_UINT8','SS_UINT16'}},'RWork',{{{'SENT_FRAMES',uint32(1)}}},'InitLevel',3,'IconTransparency','on','BlockDisplay',{{['Ethernet UDP/IP\nTX\n\nSocket ID: 0'],'center'}},'DialogFcn','rtiethernettxudpgui','BlockName',struct('Token',{{'ETHERNET_UDP_TX_BL1'}}))  RTIBlockParameters=struct('SocketIdIndex',{{2,'OFF',[1 2]}},'SocketId',{{0,'OFF',[-1 inf]}},'RemoteIp',{{['<NOT AVAILABLE>'],'OFF',[]}},'RemotePort',{{9930,'OFF',[]}},'LocalPort',{{9931,'OFF',[]}},'EnableDynamicRemoteIp',{{0,'OFF',[0 1]}},'EnableDynamicRemotePort',{{0,'OFF',[0 1]}},'FrameSize',{{'25','OFF',[1 65507]}},'EnableVariableFrameSize',{{0,'OFF',[0 1]}},'SentFramesOutPortMode',{{1,'OFF',[0 1]}},'RemoteIpNum',{{[137 148 204 55],'OFF',[0 255]}},'RemotePortNum',{{9930,'OFF',[0 65535]}},'TLCFileName',{{'rtiethernettxudp','OFF',[]}})  RTISFcnParameters=struct('SocketIdIndex','int32','SocketId','double','EnableDynamicRemoteIp','int32','EnableDynamicRemotePort','int32','FrameSize','uint16','EnableVariableFrameSize','int32','SentFramesOutPortMode','int32','RemoteIpNum','uint8','RemotePortNum','uint16','TLCFileName','char')  RTIBlockParaDefault=struct('SocketIdIndex',1,'SocketId',-1,'RemoteIp',['<NOT AVAILABLE>'],'RemotePort',['<NOT AVAILABLE>'],'LocalPort',['<NOT AVAILABLE>'],'EnableDynamicRemoteIp',0,'EnableDynamicRemotePort',0,'FrameSize',1024,'EnableVariableFrameSize',0,'SentFramesOutPortMode',1,'RemoteIpNum',[0 0 0 0],'RemotePortNum',0,'TLCFileName','rtiethernettxudp')
  UDP Send Status : Terminator
  UDP Sent Frames : Terminator
  wires:
  ETHERNET_UDP_TX_BL1/2 -> UDP Sent Frames/1
  Enable/1 -> ETHERNET_UDP_TX_BL1/2
  Send Data/1 -> ETHERNET_ENCODE_BL1/1
  ETHERNET_ENCODE_BL1/1 -> ETHERNET_UDP_TX_BL1/1
  ETHERNET_UDP_TX_BL1/1 -> UDP Send Status/1

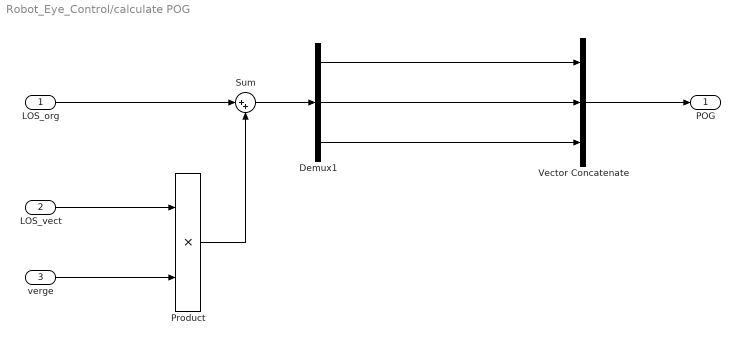
== system Robot_Eye_Control/calculate POG ==
  LOS_org : Inport
  LOS_vect : Inport  Port=2
  verge : Inport  Port=3
  Demux1 : Demux  Outputs=3
  Product : Product
  Sum : Sum  Inputs=|++
  Vector Concatenate : Concatenate  NumInputs=3  Mode=Multidimensional array  ConcatenateDimension=2
  POG : Outport
  wires:
  LOS_org/1 -> Sum/1
  Sum/1 -> Demux1/1
  Demux1/3 -> Vector Concatenate/3
  Demux1/2 -> Vector Concatenate/2
  Demux1/1 -> Vector Concatenate/1
  LOS_vect/1 -> Product/1
  Product/1 -> Sum/2
  verge/1 -> Product/2
  Vector Concatenate/1 -> POG/1

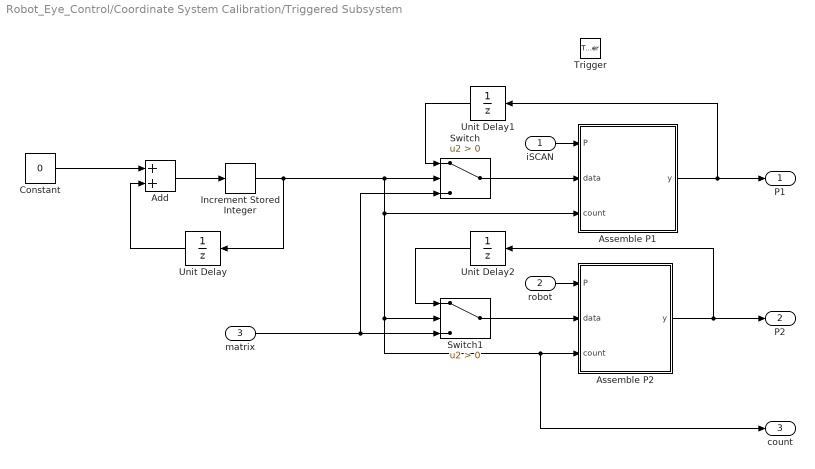
== system Robot_Eye_Control/Coordinate System Calibration/Triggered Subsystem ==
  iSCAN : Inport
  robot : Inport  Port=2
  matrix : Inport  Port=3
  Trigger : TriggerPort  VariantControl=Variant
  Add : Sum
  Assemble P1 : MATLAB Function  TreatAsAtomicUnit=on
  Assemble P2 : MATLAB Function  TreatAsAtomicUnit=on
  Constant : Constant  Value=0  VectorParams1D=off
  Increment Stored Integer : simulink/Additional Math & Discrete/Additional Math: Increment - Decrement/Increment Stored Integer
  Switch : Switch  Criteria=u2 > Threshold
  Switch1 : Switch  Criteria=u2 > Threshold
  Unit Delay : UnitDelay  SampleTime=-1
  Unit Delay1 : UnitDelay  SampleTime=-1
  Unit Delay2 : UnitDelay  SampleTime=-1
  P1 : Outport
  P2 : Outport  Port=2
  count : Outport  Port=3
  wires:
  Constant/1 -> Add/1
  Add/1 -> Increment Stored Integer/1
  Unit Delay/1 -> Add/2
  Increment Stored Integer/1 -> count/1, Assemble P2/3(count), Switch1/2, Assemble P1/3(count), Switch/2, Unit Delay/1
  matrix/1 -> Switch/3, Switch1/3
  Switch1/1 -> Assemble P2/2(data)
  robot/1 -> Assemble P2/1(P)
  iSCAN/1 -> Assemble P1/1(P)
  Switch/1 -> Assemble P1/2(data)
  Assemble P1/1(y) -> Unit Delay1/1, P1/1
  Assemble P2/1(y) -> Unit Delay2/1, P2/1
  Unit Delay1/1 -> Switch/1
  Unit Delay2/1 -> Switch1/1

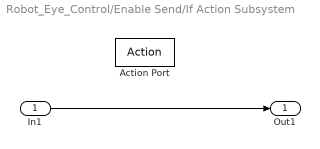
== system Robot_Eye_Control/Enable Send/If Action Subsystem ==
  In1 : Inport
  Action Port : ActionPort  ActionType=then
  Out1 : Outport
  wires:
  In1/1 -> Out1/1

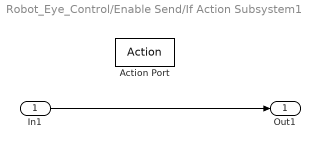
== system Robot_Eye_Control/Enable Send/If Action Subsystem1 ==
  In1 : Inport
  Action Port : ActionPort  ActionType=else
  Out1 : Outport
  wires:
  In1/1 -> Out1/1

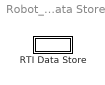
== system Robot_Eye_Control/RTI Data/RTI Data Store ==
  RTI Data Store : Subsystem  mask(RTI_DATA_STORE){}
      mask help:
      | RTI Data Store Block. This block is used by RTI to store internal model dependent data. Deleting this block will result in data loss.
      |
      | NEVER DELETE, COPY, OR MODIFY THIS BLOCK!
      mask Help:
      | RTI Data Store Block. This block is used by RTI to store internal model dependent data. Deleting this block will result in data loss.
      | 
      | NEVER DELETE, COPY, OR MODIFY THIS BLOCK!
      mask Display: text(0.5, 0.5, ' ', 'HorizontalAlignment', 'center');

== system Robot_Eye_Control/RTI Data/RTI Data Store/RTI Data Store ==
  RTI Data Store : Subsystem  mask(RTI_DATA_STORE){}
      mask help:
      | RTI Data Store Block. This block is used by RTI to store internal model dependent data. Deleting this block will result in data loss.
      |
      | NEVER DELETE, COPY, OR MODIFY THIS BLOCK!
      mask Help:
      | RTI Data Store Block. This block is used by RTI to store internal model dependent data. Deleting this block will result in data loss.
      | 
      | NEVER DELETE, COPY, OR MODIFY THIS BLOCK!
      mask Display: text(0.5, 0.5, ' ', 'HorizontalAlignment', 'center');

== system Robot_Eye_Control/RTI Data/RTI Data Store/RTI Data Store/RTI Data Store ==
  RTI Data Store : Subsystem  mask(RTI_DATA_STORE){}
      mask help:
      | RTI Data Store Block. This block is used by RTI to store internal model dependent data. Deleting this block will result in data loss.
      |
      | NEVER DELETE, COPY, OR MODIFY THIS BLOCK!
      mask Help:
      | RTI Data Store Block. This block is used by RTI to store internal model dependent data. Deleting this block will result in data loss.
      | 
      | NEVER DELETE, COPY, OR MODIFY THIS BLOCK!
      mask Display: text(0.5, 0.5, ' ', 'HorizontalAlignment', 'center');

== system Robot_Eye_Control/RTI Data/RTI Data Store/RTI Data Store/RTI Data Store/RTI Data Store ==

== matlab function Robot_Eye_Control/Coordinate System Calibration/Triggered Subsystem/Assemble P1 ==
  data: P input; y output; data input; count input
function y = fcn(P, data, count)
% Inputs:
% data..................[10x3]
% count..................[1x1]

% Output:
% y.....................[10x3]

if count > 0
    data(count,:) = P;
end
y = data;

== matlab function Robot_Eye_Control/Coordinate System Calibration/transform ==
  data: P1 input; T output; P2 input; rms output
function[T,rms] = transform(P1,P2)
% Estimates rigid body pose T from marker coordinates
%
% Input:
%	P1		(N x 3 matrix) coordinates of N markers in coordinate system 1
%	P2		(N x 3 matrix) coordinates of the same markers, now measured in coordinate system 2
%
% Output:
%	T		(4x4 matrix) homogeneous transformation matrix that transforms P1 coordinates
%			to P2 coordinates (P2 = T*P1)
%	rms		(scalar, optional) rms fit error of the rigid body model: P2 = T*P1 + error
%
% Method:
%	Soderkvist I. and Wedin P.A. (1993) Determining the movements of the skeleton using
%	well-configured markers.  Journal of Biomechanics, 26:1473-1477.    

	% error checking
	[nmarkers,ndim1]=size(P1);
	[nmarkers2,ndim2]=size(P2);
	if (ndim1 ~= 3) || (ndim2 ~= 3)
		error('hmc3_soder: matrix with marker coordinates must have 3 columns (x,y,z)');
	end
	if (nmarkers2 ~= nmarkers)
		error('hmc3+soder: matrices with marker coordinates must have same number of rows');
    end
		
	% construct matrices A and B, subtract the mean so there is only rotation
	m1=mean(P1);
	m2=mean(P2);
    A = zeros(size(P1));
    B = zeros(size(P2));
	for i=1:nmarkers
	  A(i,:)=P1(i,:)-m1;
	  B(i,:)=P2(i,:)-m2;
	end
	A = A';
	B = B';

	% The singular value decomposition to calculate rotation matrix R
	C=B*A';
	[P,~,Q]=svd(C);
	R=P*diag([1 1 det(P*Q')])*Q';

	% Calculate the translation vector from the centroid of all markers
	d=m2'-R*m1';

	% combine them into a 4x4 matrix
	T = [R d ; 0 0 0 1];

	% calculate RMS value of residuals
	sumsq = 0;
	for i=1:nmarkers
	  P2model = R*P1(i,:)' + d;
	  sumsq = sumsq + norm(P2model-P2(i,:)')^2;
	end
	rms = sqrt(sumsq/3/nmarkers);
end

== matlab function Robot_Eye_Control/decode serial data ==
  data: byteStream input; LOS_org output; LOS_vect output; verge output
function [LOS_org, LOS_vect, verge] = decode(byteStream)
values = zeros(((length(byteStream)-2)/2),1);
ii = 1;
byteStream = cast(byteStream, 'double');
    for i = 3:2:length(byteStream)
        if 0.0 <= byteStream(i+1) && byteStream(i+1) <= 20.0
            values(ii,1) = (byteStream(i+1)*255.0 + byteStream(i))/10.0;
        elseif 253.0 <= byteStream(i+1) && byteStream(i+1) <= 255.0
            values(ii,1) = ((255.0-byteStream(i+1))*255.0 + 255.0-byteStream(i))/-10.0;
        end
        ii = ii+1;
    end
    LOS_org = [values(1); values(2); values(3)];
    LOS_vect = [values(4); values(5); values(6)];
    verge = values(7);
end

== matlab function Robot_Eye_Control/Coordinate System Calibration/Triggered Subsystem/Assemble P2 ==
  data: P input; y output; data input; count input
function y = fcn(P, data, count)
% Inputs:
% data..................[10x3]
% count..................[1x1]

% Output:
% y.....................[10x3]

if count > 0
    data(count,:) = P;
end
y = data;
